simulink model "harder_m"  (Simulink 7.9)
settings: Solver=ode23tb  StartTime=0.0  StopTime=24*3600  RelTol=1e-3
values from neighbouring files (symbols this model uses):
  U = st_Varia('LongNames')    [harder_i.m]    (also in irocon_i.m; irofil_i.m)
  x0 = x0    [harder_s.m]    (also in irocon_i.m = [zeros((P.NumCel),1); zeros((P.NumCel),1); 0.3*ones(1*(P.Num; irocon_s.m; irofil_i.m = [zeros(2*(P.NumCel),1); 10*ones(2*(P.NumCel),1); 61*3*ones(1; irofil_s.m)
undefined symbols (not defined in the file or in its folder): B
settings Model: Creator=M.Sparnaaij  LastModifiedBy=M.Sparnaaij  ExtModeTrigMode=oneshot  ExtModeArmWhenConnect=off
settings DataIOCC: LimitDataPoints=off  SignalLoggingName=sigsOut
settings OptimizationCC: BooleanDataType=off
settings DebuggingCC: SaveWithParameterizedLinksMsg=none  SignalResolutionControl=TryResolveAllWithWarning  SolverPrmCheckMsg=none  MultiTaskDSMMsg=warning  MultiTaskCondExecSysMsg=none  StrictBusMsg=None
settings HardwareCC: TargetUnknown=on
settings RTWCC: IncludeERTFirstTime=on
settings GRTTargetCC: CombineOutputUpdateFcns=off  GRTInterface=on

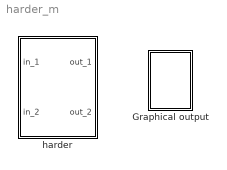
== system harder_m ==
  Graphical output : Subsystem
      settings: OpenFcn=harder_g
      mask Display:
      | plot(0,0,100,100,[80,20,20],[20,20,80],[80,69,60,52,45,39,33,28,24,20],[65,65,64,61,57,52,45,37,30,20])
      | disp('');
      | text(100,100,'harder', 'horizontalAlignment', 'right', 'verticalAlignment', 'top');
  harder : Subsystem  Description=This model calculates the removal of suspended solids with a single media filter.
      mask init:
      | filenaam='.\StimelaData\Single_media_filter1.mat';
      | 
      | errstr = st_UniqName(filenaam,'filenaam=''','SubSystem','OpenFcn');
      | if errstr, error([errstr 'The filename "' filenaam '" is already in use. Choose a different filename.']), end
      | 
      | P = harder_p(filenaam);
      | [B,x0,U]=harder_i(filenaam);
      settings: OpenFcn=|
      | filenaam='.\StimelaData\Single_media_filter1.mat';
      | st_ParameterInput('init',gcb,filenaam,'harder');
      mask Display: plot(0,0,100,100,[25.000000,25.000000,75.000000,75.000000,87.500000],[75.000000,25.000000,25.000000,30.000000,30.000000],[87.500000,75.000000,75.000000],[37.500000,37.500000,75.000000],[25.000000,75.000000],[65.000000,65.000000],[25.000000,75.000000],[42.500000,42.500000],[37.500000,42.500000],[52.500000,52.500000],[50.000000,55.000000],[52.500000,52.500000],[62.500000,67.500000],[52.500000,52.500000])

== system harder_m/Graphical output ==
  note: plotten

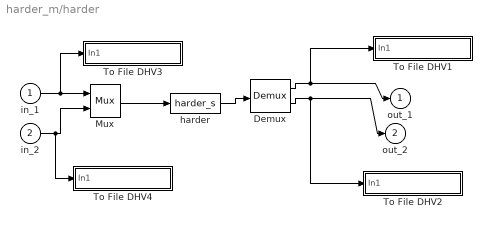
== system harder_m/harder ==
  in_1 : Inport
  in_2 : Inport  Port=2
  Demux : Demux  Outputs=[U.Number B.Measurements]
  Mux : Mux  Inputs=[U.Number B.Setpoints]
  To File DHV1 : Subsystem  mask(To File DHV){naam=[filenaam(1:length(filenaam)-4) '_out.sti']}
      mask prompts: naam "Naam van bestand"
      mask init:
      | set_param([gcb '/To File'],'Filename',naam);
      mask Display: disp(naam)
  To File DHV2 : Subsystem  mask(To File DHV){naam=[filenaam(1:length(filenaam)-4) '_EM.sti']}
      mask prompts: naam "Naam van bestand"
      mask init:
      | set_param([gcb '/To File'],'Filename',naam);
      mask Display: disp(naam)
  To File DHV3 : Subsystem  mask(To File DHV){naam=[filenaam(1:length(filenaam)-4) '_in.sti']}
      mask prompts: naam "Naam van bestand"
      mask init:
      | set_param([gcb '/To File'],'Filename',naam);
      mask Display: disp(naam)
  To File DHV4 : Subsystem  mask(To File DHV){naam=[filenaam(1:length(filenaam)-4) '_ES.sti']}
      mask prompts: naam "Naam van bestand"
      mask init:
      | set_param([gcb '/To File'],'Filename',naam);
      mask Display: disp(naam)
  harder : S-Function  FunctionName=harder_s  Parameters=B,x0,U,P  EnableBusSupport=off
  out_1 : Outport  InitialOutput=0
  out_2 : Outport  Port=2  InitialOutput=0
  wires:
  in_2/1 -> To File DHV4/1(In1), Mux/2
  Mux/1 -> harder/1
  in_1/1 -> To File DHV3/1(In1), Mux/1
  harder/1 -> Demux/1
  Demux/1 -> To File DHV1/1(In1), out_1/1
  Demux/2 -> To File DHV2/1(In1), out_2/1

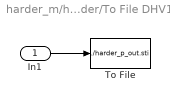
== system harder_m/harder/To File DHV1 ==
  In1 : Inport
  To File : ToFile  Filename=./harder_p_out.sti  MatrixName=harderout
  wires:
  In1/1 -> To File/1

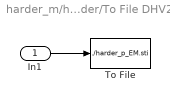
== system harder_m/harder/To File DHV2 ==
  In1 : Inport
  To File : ToFile  Filename=./harder_p_EM.sti  MatrixName=harderEM
  wires:
  In1/1 -> To File/1

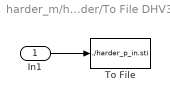
== system harder_m/harder/To File DHV3 ==
  In1 : Inport
  To File : ToFile  Filename=./harder_p_in.sti  MatrixName=harderin
  wires:
  In1/1 -> To File/1

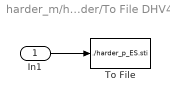
== system harder_m/harder/To File DHV4 ==
  In1 : Inport
  To File : ToFile  Filename=./harder_p_ES.sti  MatrixName=harderES
  wires:
  In1/1 -> To File/1
